simulink model "model_simulink"  (Simulink 8.4)
settings: Solver=ode45  StartTime=0.0  StopTime=200.0  RelTol=1e-3
settings Model: Creator=shaza  LastModifiedBy=Home
settings DebuggingCC: FcnCallInpInsideContextMsg=EnableAllAsWarning

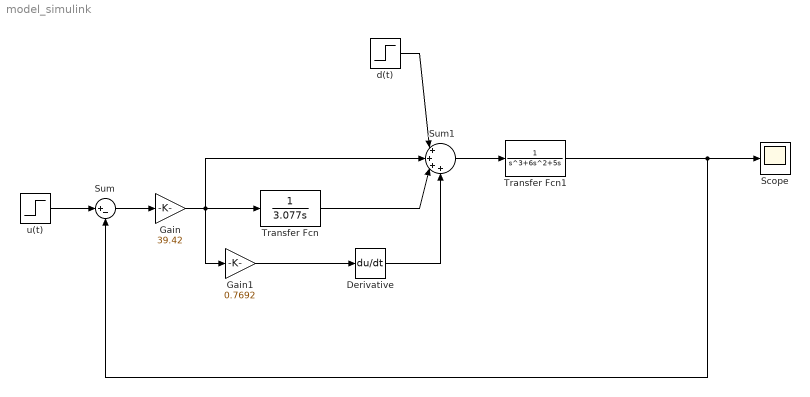
== system model_simulink ==
  Derivative : Derivative
  Gain : Gain  Gain=39.42
  Gain1 : Gain  Gain=0.7692
  Scope : Scope
  Sum : Sum  Inputs=|+-
  Sum1 : Sum  Inputs=|++++
  Transfer Fcn : TransferFcn  Denominator=[3.077 0]
  Transfer Fcn1 : TransferFcn  Denominator=[1 6 5 0]
  d(t) : Step  After=0.1  SampleTime=0
  u(t) : Step  SampleTime=0
  wires:
  u(t)/1 -> Sum/1
  Transfer Fcn1/1 -> Sum/2, Scope/1
  Gain/1 -> Sum1/2, Gain1/1, Transfer Fcn/1
  Transfer Fcn/1 -> Sum1/3
  Sum/1 -> Gain/1
  Sum1/1 -> Transfer Fcn1/1
  Gain1/1 -> Derivative/1
  Derivative/1 -> Sum1/4
  d(t)/1 -> Sum1/1
